simulink model "GCSMAVLink"  (R2026a)
settings: configuration reference "quad_config" (kept outside this file)
undefined symbols (not defined in the file): landTime, ts_uav
libraries: uavmavlinklib x2
settings Model: DataDictionary=QuadData.sldd  Creator=The MathWorks, Inc.  LastModifiedBy=The MathWorks, Inc.
settings ConfigSetRef: SourceName=quad_config

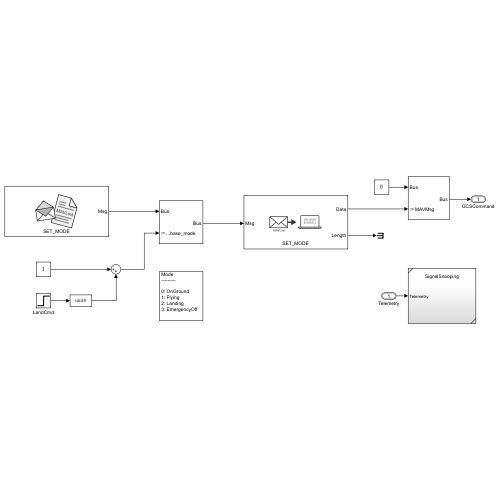
[thumbnail: Simulink's stored preview of the top-level diagram]
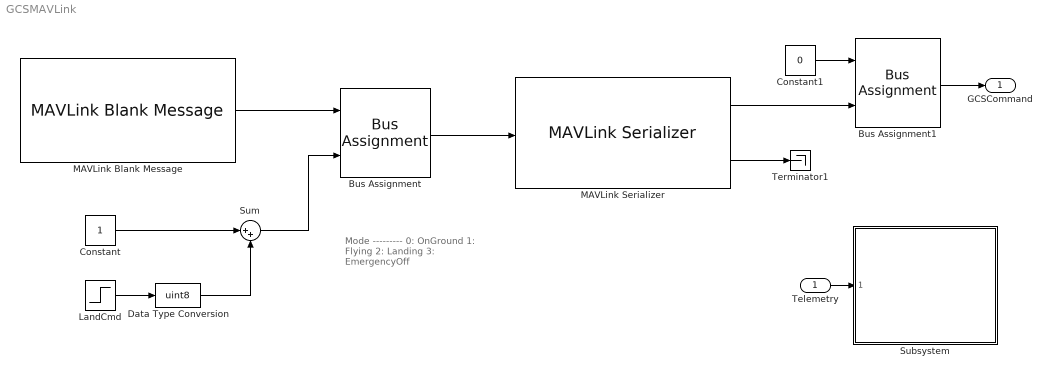
== system GCSMAVLink ==
  note: Mode
      | ---------
      |
      | 0: OnGround
      | 1: Flying
      | 2: Landing
      | 3: EmergencyOff
  Telemetry : Inport  OutDataTypeStr=Bus: Telemetry  BusOutputAsStruct=on
  Bus Assignment : BusAssignment  AssignedSignals=Payload.base_mode
  Bus Assignment1 : BusAssignment  AssignedSignals=MAVMsg
  Constant : Constant  OutDataTypeStr=uint8
  Constant1 : Constant  Value=0  OutDataTypeStr=Bus: GCSCmds
  Data Type Conversion : DataTypeConversion  OutDataTypeStr=uint8  SaturateOnIntegerOverflow=off  RndMeth=Floor
  LandCmd : Step  Time=landTime  SampleTime=ts_uav
  MAVLink Blank Message : uavmavlinklib/MAVLink Blank Message  dialectSource=Select from standard MAVLink dialects  dialect=common.xml  dialectCustom=common.xml  version=2  messageType=SET_MODE  SystemID=1  ComponentID=1  SampleTime=-1
  MAVLink Serializer : uavmavlinklib/MAVLink Serializer  dialectSource=Select from standard MAVLink dialects  dialect=common.xml  dialectCustom=common.xml  version=2  messageType=SET_MODE
  Subsystem : Subsystem  ReferencedSubsystem=SignalSnooping
  Sum : Sum  Inputs=|++
  Terminator1 : Terminator
  GCSCommand : Outport  OutDataTypeStr=Bus: GCSCmds
  wires:
  MAVLink Serializer/2 -> Terminator1/1
  Bus Assignment/1 -> MAVLink Serializer/1
  LandCmd/1 -> Data Type Conversion/1
  MAVLink Blank Message/1 -> Bus Assignment/1
  Constant/1 -> Sum/1
  Data Type Conversion/1 -> Sum/2
  Sum/1 -> Bus Assignment/2
  Bus Assignment1/1 -> GCSCommand/1
  MAVLink Serializer/1 -> Bus Assignment1/2
  Constant1/1 -> Bus Assignment1/1
  Telemetry/1 -> Subsystem/1
